simulink model "integration_on_android"  (R2019b)
settings: configuration reference "Configuration" (kept outside this file)
libraries: androidaudiovideolib x1, androiduilib x1, androidcommunicationlib x1
settings Model: DataDictionary=integration_on_android_DATA.sldd  Creator=odufour  LastModifiedBy=odufour
settings ConfigSetRef: SourceName=Configuration

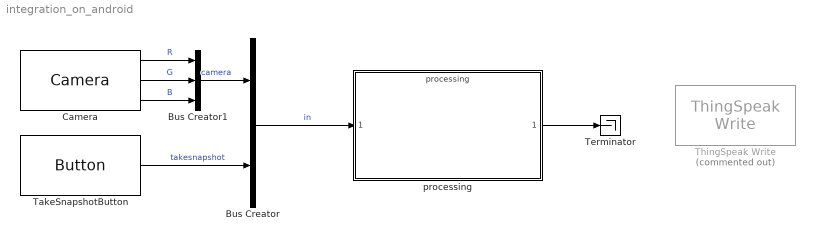
== system integration_on_android ==
  Bus Creator : BusCreator  Inputs=2  OutDataTypeStr=Bus: processing_IN  NonVirtualBus=on
  Bus Creator1 : BusCreator  Inputs=3  OutDataTypeStr=Bus: BUS_IMAGE  NonVirtualBus=on
  Camera : androidaudiovideolib/Camera  CameraLocation=Back  CameraResolutions=Back - 640x480  Width=640  Height=480  SampleTime=0.1  BlockPlatform=Android
      settings: SourceProductName=Simulink Support Package for Android Devices  SourceProductBaseCode=ANDROID
  TakeSnapshotButton : androiduilib/Button  ButtonState=Pressed  ButtonId=integration_on_android/TakeSnapshotButton  State=on  SampleTime=0.1  BlockPlatform=Android
      settings: SourceProductName=Simulink Support Package for Android Devices  SourceProductBaseCode=ANDROID
  Terminator : Terminator
  ThingSpeak Write : androidcommunicationlib/ThingSpeak Write  Commented=on  ChannelID=12345  WriteAPIKey=<Enter the write API key for your channel>  NumberOfFields=1  UpdateInterval=60  LocationEnabled=off  LocationSource=Block dialog  BlockPlatform=Android
      settings: SourceProductName=Simulink Support Package for Android Devices  SourceProductBaseCode=ANDROID
  processing : ModelReference  ModelNameDialog=processing  SimulationMode=Normal  ModelReferenceVersion=1.5
  wires:
  Camera/1 -> Bus Creator1/1  "R"
  Camera/2 -> Bus Creator1/2  "G"
  Camera/3 -> Bus Creator1/3  "B"
  Bus Creator1/1 -> Bus Creator/1  "camera"
  TakeSnapshotButton/1 -> Bus Creator/2  "takesnapshot"
  Bus Creator/1 -> processing/1  "in"
  processing/1 -> Terminator/1
